simulink model "BallandBeamControlSystem"  (R2022a)
settings: Solver=VariableStepAuto  StartTime=0.0  StopTime=10.0  RelTol=1e-3
libraries: simulink x1, slpidlib x1
settings Model: PacingRate=0.400000  Creator=ebert  LastModifiedBy=ebert

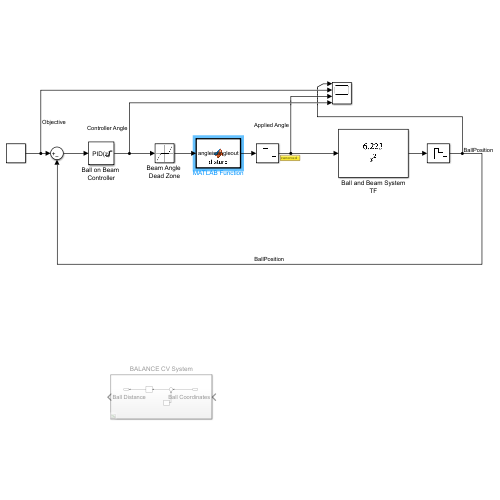
[thumbnail: Simulink's stored preview of the top-level diagram]
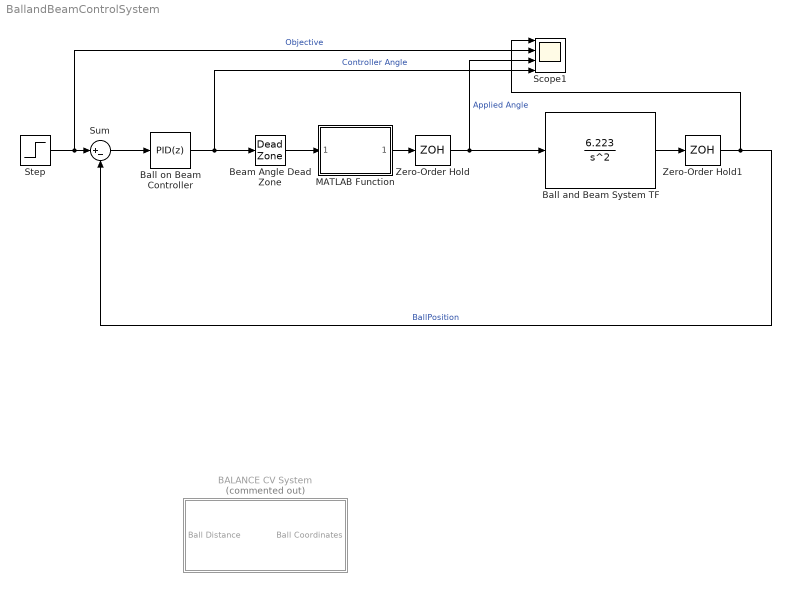
== system BallandBeamControlSystem ==
  BALANCE CV System : Subsystem  Commented=on
  Ball and Beam System TF : TransferFcn  Numerator=[6.223]  Denominator=[1 0 0]
  Ball on Beam Controller : slpidlib/PID Controller  Controller=PID  Form=Parallel  TimeDomain=Discrete-time  UseExternalTs=off  SampleTime=1/30  IntegratorMethod=Forward Euler  FilterMethod=Forward Euler  ControllerParametersSource=internal  P=0.590675028907193  I=0.0151845736692771  UseKiTs=off  D=0.456410632015891  N=2.85767184645159  UseFilter=on  TunerSelectOption=Transfer Function Based (PID Tuner App)  InitialConditionSource=internal  InitialConditionForIntegrator=0  InitialConditionForFilter=0  DifferentiatorICPrevScaledInput=0  ExternalReset=none  TrackingMode=off  Kt=1  LimitOutput=on  SatLimitsSource=internal  UpperSaturationLimit=0.3  LowerSaturationLimit=-0.3  LinearizeAsGain=off  AntiWindupMode=clamping  Kb=1  POutMin=[]  POutMax=[]  IOutMin=[]  IOutMax=[]  DOutMin=[]  DOutMax=[]  NOutMin=[]  NOutMax=[]  SumOutMin=[]  SumOutMax=[]  SaturationOutMin=[]  SaturationOutMax=[]  PParamMin=[]  PParamMax=[]  IParamMin=[]  IParamMax=[]  DParamMin=[]  DParamMax=[]  NParamMin=[]  NParamMax=[]  KbParamMin=[]  KbParamMax=[]  KtParamMin=[]  KtParamMax=[]  KbOutMin=[]  KbOutMax=[]  KtOutMin=[]  KtOutMax=[]  IntegratorOutMin=[]  IntegratorOutMax=[]  FilterOutMin=[]  FilterOutMax=[]  SumI1OutMin=[]  SumI1OutMax=[]  SumI2OutMin=[]  SumI2OutMax=[]  SumI3OutMin=[]  SumI3OutMax=[]  SumI4OutMin=[]  SumI4OutMax=[]  SumDOutMin=[]  SumDOutMax=[]  DifferentiatorOutMin=[]  DifferentiatorOutMax=[]  FilterDiffOutCoefMin=[]  FilterDiffOutCoefMax=[]  ReciprocalOutMin=[]  ReciprocalOutMax=[]  SumDenOutMin=[]  SumDenOutMax=[]  SumNumOutMin=[]  SumNumOutMax=[]  DivideOutMin=[]  DivideOutMax=[]  UdiffTsProdOutMin=[]  UdiffTsProdOutMax=[]  NTsProdOutMin=[]  NTsProdOutMax=[]  UintegralTsProdOutMin=[]  UintegralTsProdOutMax=[]  UngainTsProdOutMin=[]  UngainTsProdOutMax=[]  IntegratorContinuousStateAttributes=''  IntegratorStateMustResolveToSignalObject=off  IntegratorRTWStateStorageClass=Auto  FilterContinuousStateAttributes=''  FilterStateMustResolveToSignalObject=off  FilterRTWStateStorageClass=Auto  ParallelPVariant=InternalParameters  IdealPVariant=Disabled  IVariant=InternalParameters  DVariant=InternalParameters  IntegratorVariant=Discrete  SatVariant=Enabled  AWVariant=DiscClampingParallel  PCopyVariant=Disabled  TRVariant=Disabled  FdbkBlocksVariant=Forward  IdealPFdbkVariant=Disabled  SatFdbkVariant=Disabled  DerivativeFilterVariant=ForwardEulerFilter  NVariant=InternalParameters  NCopyVariant=Disabled  FilterICVariant=InternalICsFilter  IntegratorICVariant=InternalICs  ExternalResetVariant=Disabled  TRSumVariant=Passthrough  SumFdbkVariant=Disabled  SumVariant=Sum_PID  TsampFilterVariant=InternalTs  TsampNgainVariant=Passthrough  TsampIntegralVariant=Passthrough  ExternalSaturationOutDataTypeStr=Inherit: Same as second input  aMode=0
  Beam Angle Dead Zone : DeadZone  LowerValue=-0.01  UpperValue=0.01
  MATLAB Function : MATLAB Function  TreatAsAtomicUnit=on
  Scope1 : Scope  NumInputPorts=4
  Step : Step  Time=0  After=0.173  SampleTime=0
  Sum : Sum  Inputs=|+-
  Zero-Order Hold : ZeroOrderHold  SampleTime=-1
  Zero-Order Hold1 : ZeroOrderHold  SampleTime=-1
  wires:
  Ball on Beam Controller/1 -> Scope1/4, Beam Angle Dead Zone/1  "Controller Angle"
  Step/1 -> Scope1/2, Sum/1  "Objective"
  Ball and Beam System TF/1 -> Zero-Order Hold1/1
  Beam Angle Dead Zone/1 -> MATLAB Function/1(anglein)
  Sum/1 -> Ball on Beam Controller/1
  Zero-Order Hold1/1 -> Scope1/1, Sum/2  "BallPosition"
  Zero-Order Hold/1 -> Ball and Beam System TF/1, Scope1/3  "Applied Angle"
  MATLAB Function/1(angleout) -> Zero-Order Hold/1

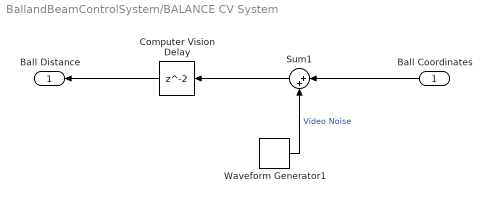
== system BallandBeamControlSystem/BALANCE CV System ==
  Ball Coordinates : Inport
  Computer Vision Delay : Delay
  Sum1 : Sum  Inputs=|++
  Waveform Generator1 : simulink/Sources/Waveform Generator  OutMin=[]  OutMax=[]  OutDataTypeStr=double  SelectedSignal=1  Signals=sin(0.0001,3,1)  BlockNames=MultiportSwitch_425a7e8e9f63443  SampleTime=0.1
  Ball Distance : Outport
  wires:
  Waveform Generator1/1 -> Sum1/2  "Video Noise"
  Sum1/1 -> Computer Vision Delay/1
  Computer Vision Delay/1 -> Ball Distance/1
  Ball Coordinates/1 -> Sum1/1

== matlab function BallandBeamControlSystem/MATLAB Function ==
  data: anglein input; angleout output
function angleout = disturb(anglein)

if(abs(anglein)<0.01 && abs(anglein)>0.001)
    angleout=sign(anglein)*0.01;
else
    angleout=anglein;
end
end
